simulink model "test1"  (R2020b)
settings: Solver=VariableStepAuto  StartTime=0.0  StopTime=10.0  RelTol=1e-3
libraries: aerolibatmos2 x1, aerolibasang x1
settings Model: Creator=simon  LastModifiedBy=simon

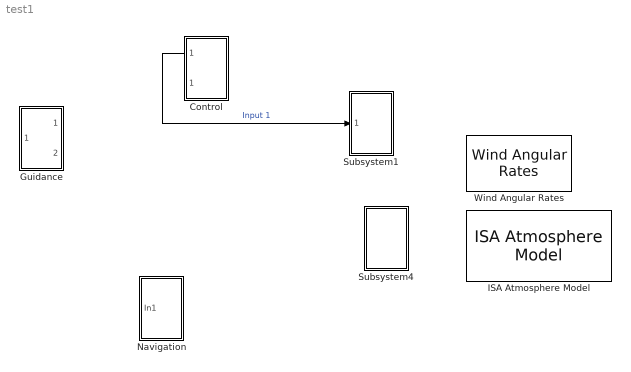
== system test1 ==
  Control : Subsystem
      settings: PortSchema="{\"entries\":[{\"content\":{\"sides\":[{\"content\":{\"connectorIds\":[\"Out1\",\"In1\"]},\"type\":\"ConnectorPlacement.EquallySpacedRectSide\",\"uuid\":\"ac5cbbab-1d56-4618-9258-c47c90f82337\"},{\"content\":{\"connectorIds\":[],\"side\":\"RIGHT\"},\"type\":\"ConnectorPlacement.EquallySpacedRectSide\",\"uuid\":\"2cf9efa2-7fb6-4524-9ce3-c515f971457d\"},{\"content\":{\"connectorIds\":[],\"side\":\"TOP\"},\"type\":\"ConnectorPlacement.EquallySpacedRectSide\",\"uuid\":\"b3910ae6-2871-4c23-9b6a-6783629c3ab5\"},{\"content\":{\"connectorIds\":[],\"side\":\"HIDDEN\"},\"type\":\"ConnectorPlacement.EquallySpacedRectSide\",\"uuid\":\"1f32bb7a-d51f-4b04-99be-963d3396ffc6\"}]},\"type\":\"ConnectorPlacement.EquallySpacedConnector\",\"uuid\":\"9c0430b5-3be8-4c08-bfe0-edf7b6f6e980\"}],\"packageUris\":[\"http://schema.mathworks.com/mf0/Connector/R2020b\"],\"version\":\"1.0\"}"
  Guidance : Subsystem
  ISA Atmosphere Model : aerolibatmos2/ISA Atmosphere Model  custom=off  g=9.80665  gamma=1.4  R=287.0531  L=0.0065  h_trop=11000  h_strat=20000  rho0=1.225  P0=101325  T0=288.15  h0=0
  Navigation : Subsystem
  Subsystem1 : Subsystem
  Subsystem4 : Subsystem
  Wind Angular Rates : aerolibasang/Wind Angular Rates
      settings: SourceProductBaseCode=AE
  wires:
  Control/1(Output1) -> Subsystem1/1(Input 1)  "Input 1"

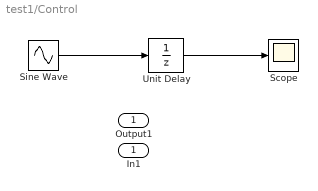
== system test1/Control ==
  In1 : Inport
  Scope : Scope
  Sine Wave : Sin  SampleTime=0
  Unit Delay : UnitDelay  SampleTime=-1  HasFrameUpgradeWarning=on
  Output1 : Outport
  wires:
  Unit Delay/1 -> Scope/1
  Sine Wave/1 -> Unit Delay/1

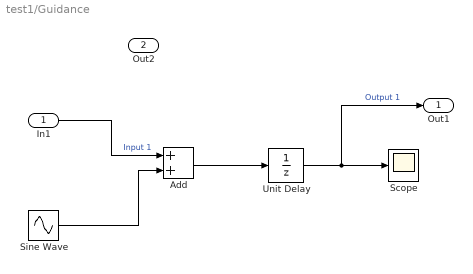
== system test1/Guidance ==
  In1 : Inport
  Add : Sum
  Scope : Scope
  Sine Wave : Sin  SampleTime=0
  Unit Delay : UnitDelay  SampleTime=-1  HasFrameUpgradeWarning=on
  Out1 : Outport
  Out2 : Outport  Port=2
  wires:
  Unit Delay/1 -> Out1/1, Scope/1  "Output 1"
  Sine Wave/1 -> Add/2
  Add/1 -> Unit Delay/1
  In1/1 -> Add/1  "Input 1"

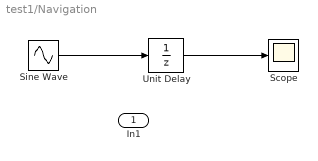
== system test1/Navigation ==
  In1 : Inport
  Scope : Scope
  Sine Wave : Sin  SampleTime=0
  Unit Delay : UnitDelay  SampleTime=-1  HasFrameUpgradeWarning=on
  wires:
  Unit Delay/1 -> Scope/1
  Sine Wave/1 -> Unit Delay/1

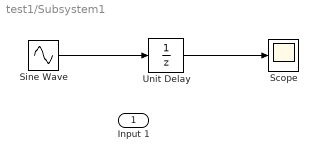
== system test1/Subsystem1 ==
  Input 1 : Inport
  Scope : Scope
  Sine Wave : Sin  SampleTime=0
  Unit Delay : UnitDelay  SampleTime=-1  HasFrameUpgradeWarning=on
  wires:
  Unit Delay/1 -> Scope/1
  Sine Wave/1 -> Unit Delay/1

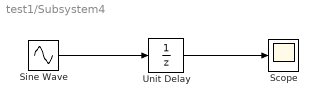
== system test1/Subsystem4 ==
  Scope : Scope
  Sine Wave : Sin  SampleTime=0
  Unit Delay : UnitDelay  SampleTime=-1  HasFrameUpgradeWarning=on
  wires:
  Unit Delay/1 -> Scope/1
  Sine Wave/1 -> Unit Delay/1
